simulink model "Observer_reconstruction"  (R2019b)
settings: Solver=ode1  StartTime=0.0  StopTime=5  FixedStep=0.002  RelTol=1e-3
values from neighbouring files (symbols this model uses):
  data = e_h.load_data    [potentiometer_recover.m]
undefined symbols (not defined in the file or in its folder): controller
settings Model: Creator=giacomo  LastModifiedBy=giacomo

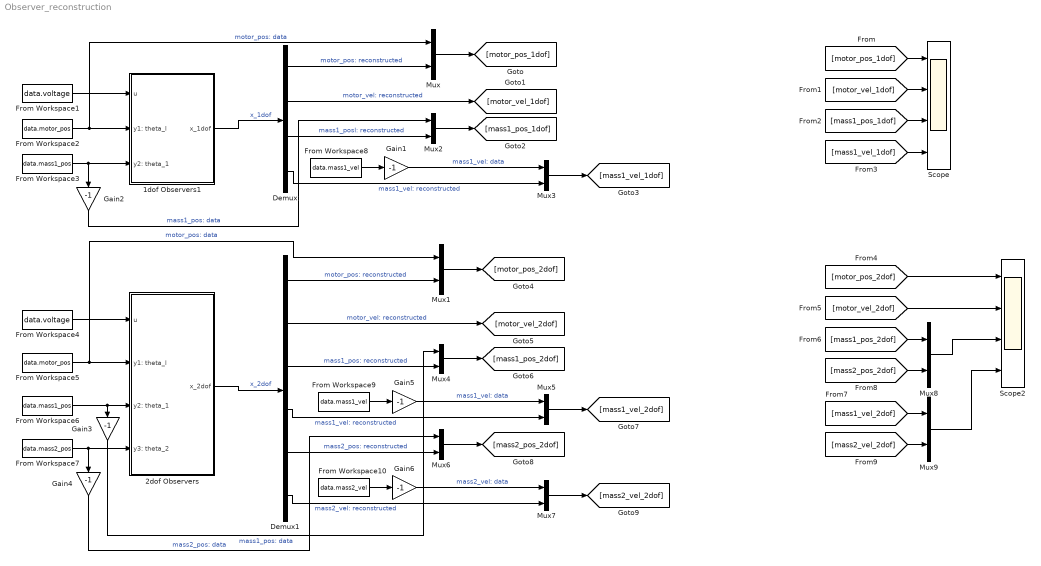
== system Observer_reconstruction ==
  1dof Observers1 : Subsystem
  2dof Observers : Subsystem
  Demux : Demux
  Demux1 : Demux  Outputs=6
  From Workspace1 : FromWorkspace  VariableName=data.voltage  SampleTime=0
  From Workspace10 : FromWorkspace  VariableName=data.mass2_vel  SampleTime=0
  From Workspace2 : FromWorkspace  VariableName=data.motor_pos  SampleTime=0
  From Workspace3 : FromWorkspace  VariableName=data.mass1_pos  SampleTime=0
  From Workspace4 : FromWorkspace  VariableName=data.voltage  SampleTime=0
  From Workspace5 : FromWorkspace  VariableName=data.motor_pos  SampleTime=0
  From Workspace6 : FromWorkspace  VariableName=data.mass1_pos  SampleTime=0
  From Workspace7 : FromWorkspace  VariableName=data.mass2_pos  SampleTime=0
  From Workspace8 : FromWorkspace  VariableName=data.mass1_vel  SampleTime=0
  From Workspace9 : FromWorkspace  VariableName=data.mass1_vel  SampleTime=0
  Gain{1..6} (6 alike) : Gain  Gain=-1
  Mux{,1..9} (10 alike) : Mux  Inputs=2
  Scope : Scope  NumInputPorts=4
  Scope2 : Scope  NumInputPorts=4
  wires:
  From Workspace2/1 -> Mux/1, 1dof Observers1/2(y1: theta_l)  "motor_pos: data"
  Demux/3 -> Mux2/2  "mass1_posl: reconstructed"
  1dof Observers1/1(x_1dof) -> Demux/1  "x_1dof"
  From Workspace1/1 -> 1dof Observers1/1(u)
  Demux/1 -> Mux/2  "motor_pos: reconstructed"
  Demux/4 -> Mux3/2  "mass1_vel: reconstructed"
  Mux/1 -> [motor_pos_1dof]
  Gain1/1 -> Mux3/1  "mass1_vel: data"
  From Workspace3/1 -> 1dof Observers1/3(y2: theta_1), Gain2/1
  Gain2/1 -> Mux2/1  "mass1_pos: data"
  [motor_pos_1dof] -> Scope/1
  Demux/2 -> [motor_vel_1dof]  "motor_vel: reconstructed"
  [motor_vel_1dof] -> Scope/2
  Mux2/1 -> [mass1_pos_1dof]
  Mux3/1 -> [mass1_vel_1dof]
  [mass1_pos_1dof] -> Scope/3
  [mass1_vel_1dof] -> Scope/4
  From Workspace8/1 -> Gain1/1
  From Workspace4/1 -> 2dof Observers/1("u ")
  From Workspace6/1 -> 2dof Observers/3(y2: theta_1), Gain3/1
  From Workspace7/1 -> 2dof Observers/4(y3: theta_2), Gain4/1
  Gain3/1 -> Mux4/1  "mass1_pos: data"
  2dof Observers/1(x_2dof) -> Demux1/1  "x_2dof"
  Mux5/1 -> [mass1_vel_2dof]
  Mux1/1 -> [motor_pos_2dof]
  From Workspace5/1 -> Mux1/1, 2dof Observers/2(y1: theta_l)  "motor_pos: data"
  Demux1/1 -> Mux1/2  "motor_pos: reconstructed"
  Demux1/3 -> Mux4/2  "mass1_pos: reconstructed"
  Demux1/4 -> Mux5/2  "mass1_vel: reconstructed"
  Mux4/1 -> [mass1_pos_2dof]
  Gain5/1 -> Mux5/1  "mass1_vel: data"
  Demux1/2 -> [motor_vel_2dof]  "motor_vel: reconstructed"
  From Workspace9/1 -> Gain5/1
  Mux7/1 -> [mass2_vel_2dof]
  Gain6/1 -> Mux7/1  "mass2_vel: data"
  From Workspace10/1 -> Gain6/1
  Demux1/5 -> Mux6/2  "mass2_pos: reconstructed"
  Demux1/6 -> Mux7/2  "mass2_vel: reconstructed"
  Mux6/1 -> [mass2_pos_2dof]
  Gain4/1 -> Mux6/1  "mass2_pos: data"
  [motor_pos_2dof] -> Scope2/1
  [motor_vel_2dof] -> Scope2/2
  [mass1_pos_2dof] -> Mux8/1
  [mass2_pos_2dof] -> Mux8/2
  Mux8/1 -> Scope2/3
  [mass2_vel_2dof] -> Mux9/2
  Mux9/1 -> Scope2/4
  [mass1_vel_2dof] -> Mux9/1

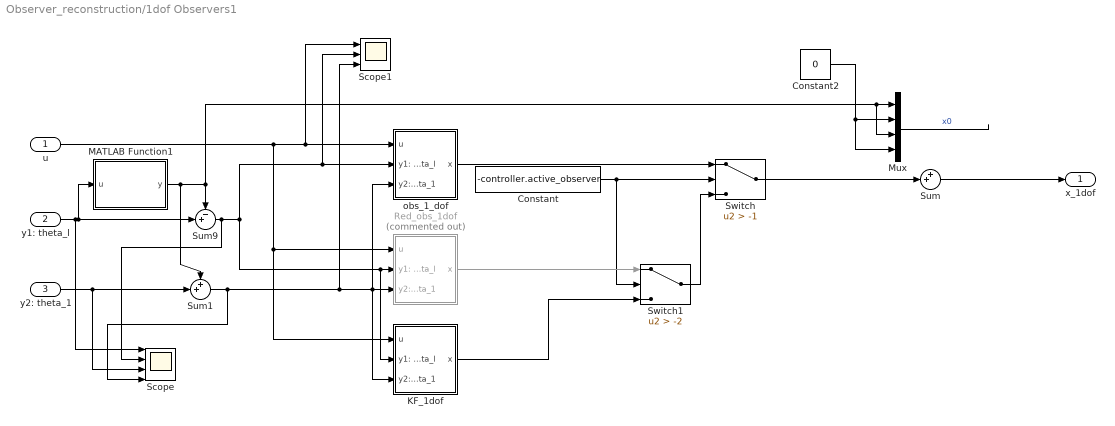
== system Observer_reconstruction/1dof Observers1 ==
  u : Inport
  y1: theta_l : Inport  Port=2
  y2: theta_1 : Inport  Port=3
  Constant : Constant  Value=-controller.active_observer
  Constant2 : Constant  Value=0
  KF_1dof : Subsystem
  MATLAB Function1 : MATLAB Function  TreatAsAtomicUnit=on  SystemSampleTime=0.002
  Mux : Mux
  Red_obs_1dof : Subsystem  Commented=on
  Scope : Scope  NumInputPorts=4
  Scope1 : Scope  NumInputPorts=3
  Sum : Sum  Inputs=++|
  Sum1 : Sum  Inputs=++|
  Sum9 : Sum  Inputs=-+|
  Switch : Switch  Criteria=u2 > Threshold  Threshold=-1
  Switch1 : Switch  Criteria=u2 > Threshold  Threshold=-2
  obs_1_dof : Subsystem
  x_1dof : Outport
  wires:
  Sum9/1 -> Scope/2, KF_1dof/2(y1: theta_l), Red_obs_1dof/2(y1: theta_l), Scope1/2, obs_1_dof/2(y1: theta_l)
  Sum1/1 -> Scope/4, Scope1/3, KF_1dof/3(y2: theta_1), obs_1_dof/3(y2: theta_1), Red_obs_1dof/3(y2: theta_1)
  Constant/1 -> Switch1/2, Switch/2
  u/1 -> Red_obs_1dof/1(u), KF_1dof/1(u), Scope1/1, obs_1_dof/1(u)
  Sum/1 -> x_1dof/1
  MATLAB Function1/1(y) -> Sum1/1, Sum9/1, Mux/3, Mux/1
  Mux/1 -> ?  "x0"
  Constant2/1 -> Mux/4, Mux/2
  Switch/1 -> Sum/2
  y1: theta_l/1 -> Scope/1, MATLAB Function1/1(u), Sum9/2
  obs_1_dof/1(x) -> Switch/1
  Red_obs_1dof/1(x) -> Switch1/1
  Switch1/1 -> Switch/3
  KF_1dof/1(x) -> Switch1/3
  y2: theta_1/1 -> Scope/3, Sum1/2

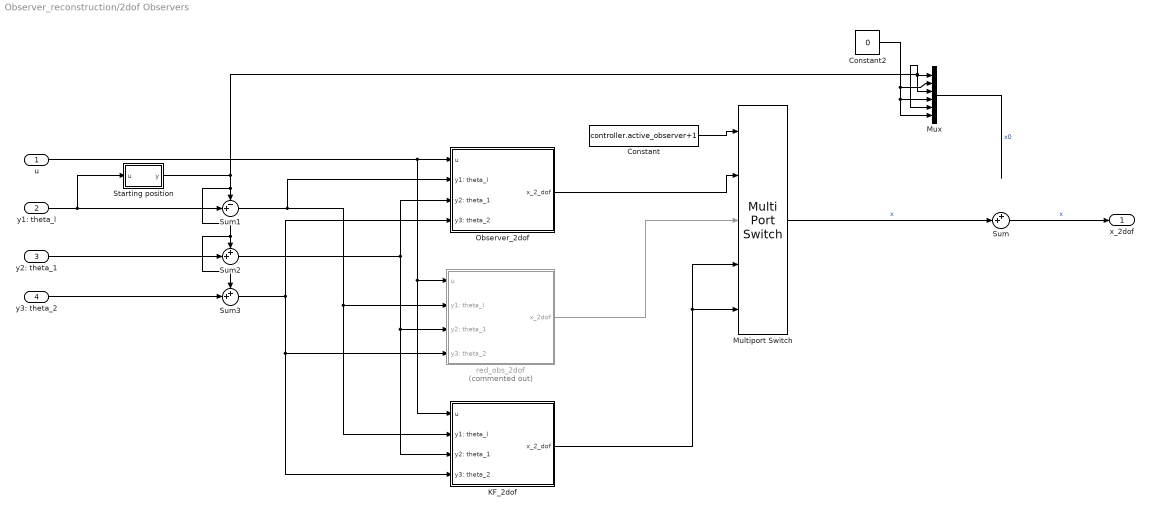
== system Observer_reconstruction/2dof Observers ==
  "u " : Inport
  y1: theta_l : Inport  Port=2
  y2: theta_1 : Inport  Port=3
  y3: theta_2 : Inport  Port=4
  Constant : Constant  Value=controller.active_observer+1
  Constant2 : Constant  Value=0
  KF_2dof : Subsystem
  Multiport Switch : MultiPortSwitch  Inputs=4
  Mux : Mux  Inputs=6
  Observer_2dof : Subsystem
  Starting position : MATLAB Function  TreatAsAtomicUnit=on  SystemSampleTime=0.002
  Sum : Sum  Inputs=++|
  Sum1 : Sum  Inputs=-+|
  Sum2 : Sum  Inputs=++|
  Sum3 : Sum  Inputs=++|
  red_obs_2dof : Subsystem  Commented=on
  x_2dof : Outport
  wires:
  Sum3/1 -> KF_2dof/4(y3: theta_2), red_obs_2dof/4(y3: theta_2), Observer_2dof/4(y3: theta_2)
  Sum2/1 -> KF_2dof/3(y2: theta_1), red_obs_2dof/3(y2: theta_1), Observer_2dof/3(y2: theta_1)
  "u "/1 -> KF_2dof/1(u), red_obs_2dof/1(u), Observer_2dof/1(u)
  Sum/1 -> x_2dof/1  "x"
  Starting position/1(y) -> Sum3/1, Sum2/1, Sum1/1, Mux/5, Mux/3, Mux/1
  Constant2/1 -> Mux/6, Mux/4, Mux/2
  Mux/1 -> ?  "x0"
  Sum1/1 -> KF_2dof/2(y1: theta_l), red_obs_2dof/2(y1: theta_l), Observer_2dof/2(y1: theta_l)
  y1: theta_l/1 -> Sum1/2, Starting position/1(u)
  Constant/1 -> Multiport Switch/1
  Observer_2dof/1(x_2_dof) -> Multiport Switch/2
  Multiport Switch/1 -> Sum/2  "x"
  y3: theta_2/1 -> Sum3/2
  y2: theta_1/1 -> Sum2/2
  red_obs_2dof/1(x_2dof) -> Multiport Switch/3
  KF_2dof/1(x_2_dof) -> Multiport Switch/5, Multiport Switch/4

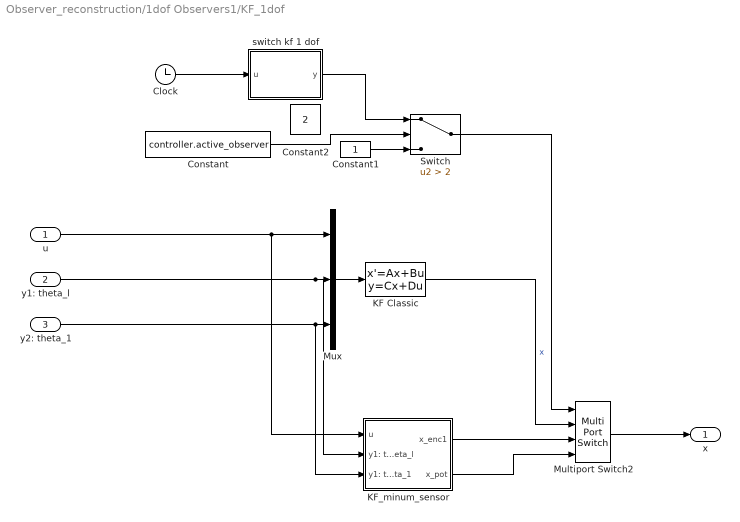
== system Observer_reconstruction/1dof Observers1/KF_1dof ==
  u : Inport
  y1: theta_l : Inport  Port=2
  y2: theta_1 : Inport  Port=3
  Clock : Clock
  Constant : Constant  Value=controller.active_observer
  Constant1 : Constant
  Constant2 : Constant  Value=2
  KF Classic : StateSpace  A=controller.KF_1dof.A  B=controller.KF_1dof.B  C=controller.KF_1dof.C  D=controller.KF_1dof.D  InitialCondition=[]
  KF_minum_sensor : Subsystem
  Multiport Switch2 : MultiPortSwitch
  Mux : Mux  Inputs=3
  Switch : Switch  Criteria=u2 > Threshold  Threshold=2
  switch kf 1 dof : MATLAB Function  TreatAsAtomicUnit=on
  x : Outport
  wires:
  Mux/1 -> KF Classic/1
  u/1 -> KF_minum_sensor/1(u), Mux/1
  y1: theta_l/1 -> KF_minum_sensor/2(y1: theta_l), Mux/2
  y2: theta_1/1 -> KF_minum_sensor/3(y1: theta_1), Mux/3
  KF Classic/1 -> Multiport Switch2/2  "x"
  Clock/1 -> switch kf 1 dof/1(u)
  Constant1/1 -> Switch/3
  switch kf 1 dof/1(y) -> Switch/1
  Constant/1 -> Switch/2
  Multiport Switch2/1 -> x/1
  KF_minum_sensor/1(x_enc1) -> Multiport Switch2/3
  KF_minum_sensor/2(x_pot) -> Multiport Switch2/4
  Switch/1 -> Multiport Switch2/1

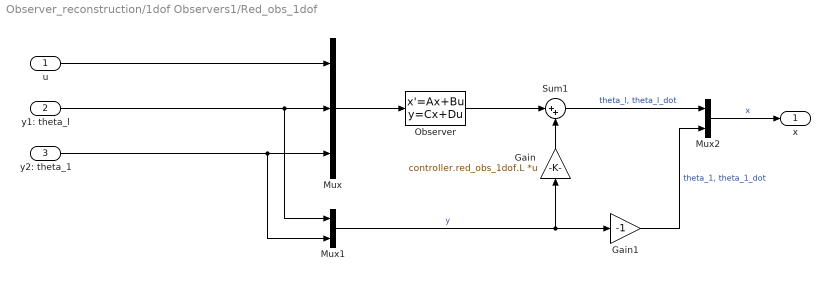
== system Observer_reconstruction/1dof Observers1/Red_obs_1dof ==
  u : Inport
  y1: theta_l : Inport  Port=2
  y2: theta_1 : Inport  Port=3
  Gain : Gain  Gain=controller.red_obs_1dof.L  Multiplication=Matrix(K*u)
  Gain1 : Gain  Gain=-1
  Mux : Mux  Inputs=3
  Mux1 : Mux  Inputs=2
  Mux2 : Mux  Inputs=2
  Observer : StateSpace  A=controller.red_obs_1dof.A  B=controller.red_obs_1dof.B  C=controller.red_obs_1dof.C  D=controller.red_obs_1dof.D  InitialCondition=[data.motor_pos_0;0]
  Sum1 : Sum  Inputs=|++
  x : Outport
  wires:
  Mux2/1 -> x/1  "x"
  u/1 -> Mux/1
  Gain1/1 -> Mux2/2  "theta_1, theta_1_dot"
  y2: theta_1/1 -> Mux/3, Mux1/2
  Gain/1 -> Sum1/2
  Mux1/1 -> Gain/1, Gain1/1  "y"
  y1: theta_l/1 -> Mux/2, Mux1/1
  Mux/1 -> Observer/1
  Sum1/1 -> Mux2/1  "theta_l, theta_l_dot"
  Observer/1 -> Sum1/1

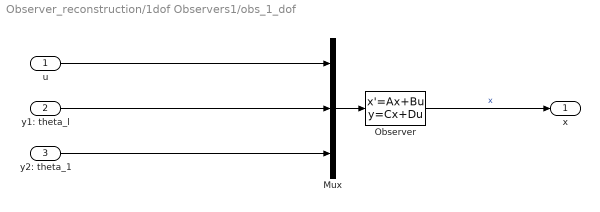
== system Observer_reconstruction/1dof Observers1/obs_1_dof ==
  u : Inport
  y1: theta_l : Inport  Port=2
  y2: theta_1 : Inport  Port=3
  Mux : Mux  Inputs=3
  Observer : StateSpace  A=controller.obs_1dof.A  B=controller.obs_1dof.B  C=controller.obs_1dof.C  D=controller.obs_1dof.D  InitialCondition=[]
  x : Outport
  wires:
  Mux/1 -> Observer/1
  u/1 -> Mux/1
  y1: theta_l/1 -> Mux/2
  y2: theta_1/1 -> Mux/3
  Observer/1 -> x/1  "x"

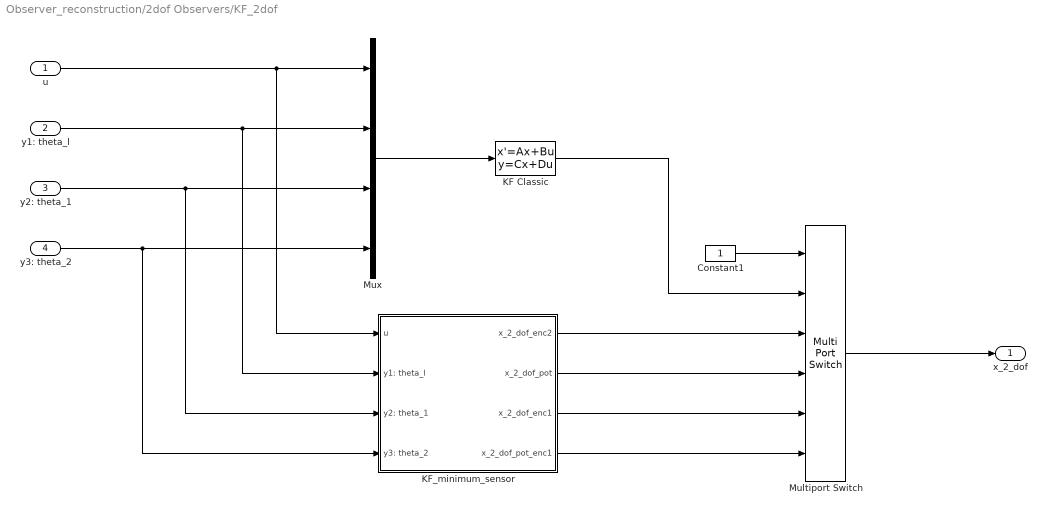
== system Observer_reconstruction/2dof Observers/KF_2dof ==
  u : Inport
  y1: theta_l : Inport  Port=2
  y2: theta_1 : Inport  Port=3
  y3: theta_2 : Inport  Port=4
  Constant1 : Constant
  KF Classic : StateSpace  A=controller.KF_2dof.A  B=controller.KF_2dof.B  C=controller.KF_2dof.C  D=controller.KF_2dof.D  InitialCondition=[]
  KF_minimum_sensor : Subsystem
  Multiport Switch : MultiPortSwitch  Inputs=5
  Mux : Mux
  x_2_dof : Outport
  wires:
  y1: theta_l/1 -> KF_minimum_sensor/2(y1: theta_l), Mux/2
  u/1 -> KF_minimum_sensor/1(u), Mux/1
  y3: theta_2/1 -> Mux/4, KF_minimum_sensor/4(y3: theta_2)
  Mux/1 -> KF Classic/1
  y2: theta_1/1 -> KF_minimum_sensor/3(y2: theta_1), Mux/3
  KF_minimum_sensor/1(x_2_dof_enc2) -> Multiport Switch/3
  KF_minimum_sensor/3(x_2_dof_enc1) -> Multiport Switch/5
  KF Classic/1 -> Multiport Switch/2
  KF_minimum_sensor/2(x_2_dof_pot) -> Multiport Switch/4
  Multiport Switch/1 -> x_2_dof/1
  KF_minimum_sensor/4(x_2_dof_pot_enc1) -> Multiport Switch/6
  Constant1/1 -> Multiport Switch/1

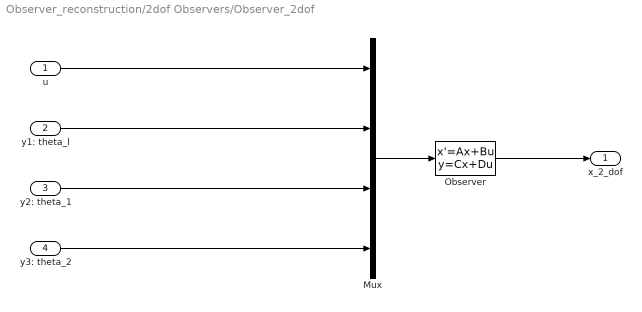
== system Observer_reconstruction/2dof Observers/Observer_2dof ==
  u : Inport
  y1: theta_l : Inport  Port=2
  y2: theta_1 : Inport  Port=3
  y3: theta_2 : Inport  Port=4
  Mux : Mux
  Observer : StateSpace  A=controller.obs_2dof.A  B=controller.obs_2dof.B  C=controller.obs_2dof.C  D=controller.obs_2dof.D  InitialCondition=[]
  x_2_dof : Outport
  wires:
  Observer/1 -> x_2_dof/1
  y1: theta_l/1 -> Mux/2
  u/1 -> Mux/1
  y3: theta_2/1 -> Mux/4
  Mux/1 -> Observer/1
  y2: theta_1/1 -> Mux/3

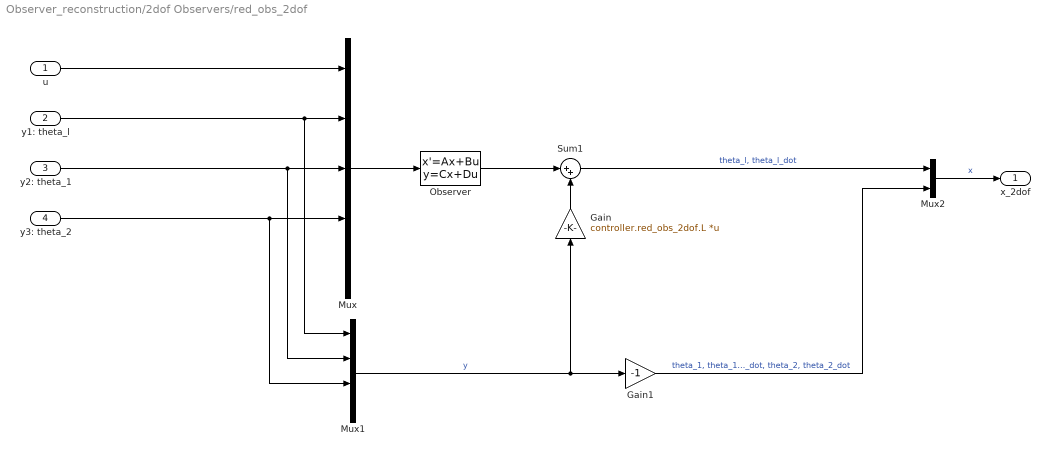
== system Observer_reconstruction/2dof Observers/red_obs_2dof ==
  u : Inport
  y1: theta_l : Inport  Port=2
  y2: theta_1 : Inport  Port=3
  y3: theta_2 : Inport  Port=4
  Gain : Gain  Gain=controller.red_obs_2dof.L  Multiplication=Matrix(K*u)
  Gain1 : Gain  Gain=-1
  Mux : Mux  Inputs=5
  Mux1 : Mux
  Mux2 : Mux  Inputs=2
  Observer : StateSpace  A=controller.red_obs_2dof.A  B=controller.red_obs_2dof.B  C=controller.red_obs_2dof.C  D=controller.red_obs_2dof.D  InitialCondition=[data.motor_pos_0;0]
  Sum1 : Sum  Inputs=|++
  x_2dof : Outport
  wires:
  Sum1/1 -> Mux2/1  "theta_l, theta_l_dot"
  y1: theta_l/1 -> Mux1/1, Mux/2
  Mux/1 -> Observer/1
  Observer/1 -> Sum1/1
  y2: theta_1/1 -> Mux1/2, Mux/3
  y3: theta_2/1 -> Mux1/3, Mux/4
  Mux1/1 -> Gain/1, Gain1/1  "y"
  u/1 -> Mux/1
  Gain/1 -> Sum1/2
  Gain1/1 -> Mux2/2  "theta_1, theta_1_dot, theta_2, theta_2_dot"
  Mux2/1 -> x_2dof/1  "x"

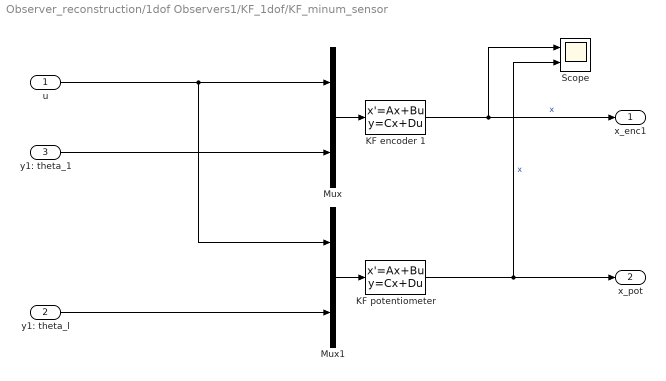
== system Observer_reconstruction/1dof Observers1/KF_1dof/KF_minum_sensor ==
  u : Inport
  y1: theta_l : Inport  Port=2
  y1: theta_1 : Inport  Port=3
  KF encoder 1 : StateSpace  A=controller.minKF_1dof_enc1.A  B=controller.minKF_1dof_enc1.B  C=controller.minKF_1dof_enc1.C  D=controller.minKF_1dof_enc1.D  InitialCondition=[]
  KF potentiometer : StateSpace  A=controller.minKF_1dof_pot.A  B=controller.minKF_1dof_pot.B  C=controller.minKF_1dof_pot.C  D=controller.minKF_1dof_pot.D  InitialCondition=[]
  Mux : Mux  Inputs=2
  Mux1 : Mux  Inputs=2
  Scope : Scope  NumInputPorts=2
  x_enc1 : Outport
  x_pot : Outport  Port=2
  wires:
  Mux/1 -> KF encoder 1/1
  y1: theta_1/1 -> Mux/2
  KF encoder 1/1 -> x_enc1/1, Scope/1  "x"
  u/1 -> Mux1/1, Mux/1
  y1: theta_l/1 -> Mux1/2
  Mux1/1 -> KF potentiometer/1
  KF potentiometer/1 -> x_pot/1, Scope/2  "x"

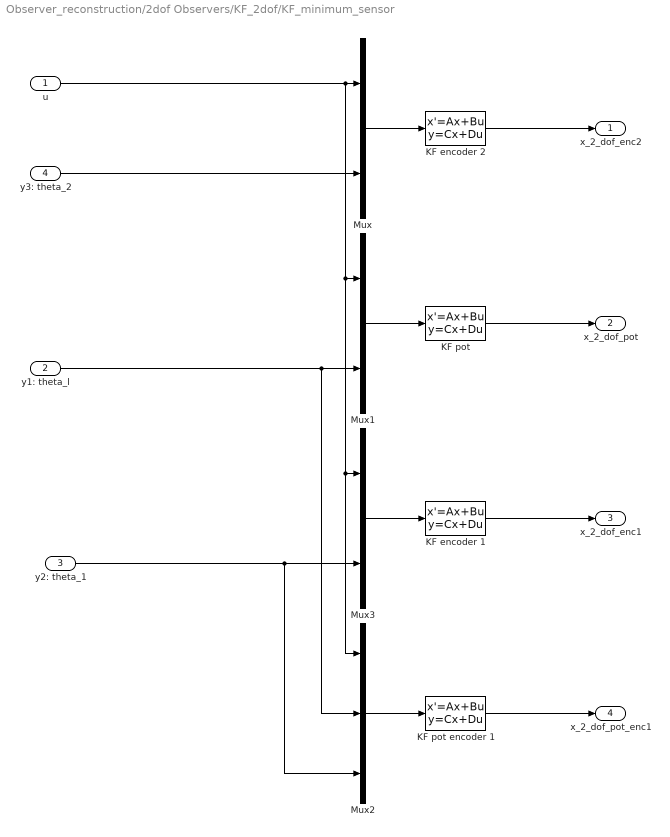
== system Observer_reconstruction/2dof Observers/KF_2dof/KF_minimum_sensor ==
  u : Inport
  y1: theta_l : Inport  Port=2
  y2: theta_1 : Inport  Port=3
  y3: theta_2 : Inport  Port=4
  KF encoder 1 : StateSpace  A=controller.minKF_2dof_enc1.A  B=controller.minKF_2dof_enc1.B  C=controller.minKF_2dof_enc1.C  D=controller.minKF_2dof_enc1.D  InitialCondition=[]
  KF encoder 2 : StateSpace  A=controller.minKF_2dof_enc2.A  B=controller.minKF_2dof_enc2.B  C=controller.minKF_2dof_enc2.C  D=controller.minKF_2dof_enc2.D  InitialCondition=[]
  KF pot : StateSpace  A=controller.minKF_2dof_pot.A  B=controller.minKF_2dof_pot.B  C=controller.minKF_2dof_pot.C  D=controller.minKF_2dof_pot.D  InitialCondition=[]
  KF pot encoder 1 : StateSpace  A=controller.minKF_2dof_potenc1.A  B=controller.minKF_2dof_potenc1.B  C=controller.minKF_2dof_potenc1.C  D=controller.minKF_2dof_potenc1.D  InitialCondition=[]
  Mux : Mux  Inputs=2
  Mux1 : Mux  Inputs=2
  Mux2 : Mux  Inputs=3
  Mux3 : Mux  Inputs=2
  x_2_dof_enc2 : Outport
  x_2_dof_pot : Outport  Port=2
  x_2_dof_enc1 : Outport  Port=3
  x_2_dof_pot_enc1 : Outport  Port=4
  wires:
  y3: theta_2/1 -> Mux/2
  u/1 -> Mux2/1, Mux3/1, Mux1/1, Mux/1
  Mux/1 -> KF encoder 2/1
  Mux2/1 -> KF pot encoder 1/1
  Mux3/1 -> KF encoder 1/1
  Mux1/1 -> KF pot/1
  y1: theta_l/1 -> Mux1/2, Mux2/2
  y2: theta_1/1 -> Mux3/2, Mux2/3
  KF encoder 2/1 -> x_2_dof_enc2/1
  KF encoder 1/1 -> x_2_dof_enc1/1
  KF pot/1 -> x_2_dof_pot/1
  KF pot encoder 1/1 -> x_2_dof_pot_enc1/1

== matlab function Observer_reconstruction/1dof Observers1/KF_1dof/switch kf 1 dof ==
  data: u input; y output
function y = fcn(u)
if u < 15
    % kf classic
    y = 1;
elseif u <30 
    % kf enc 1
    y = 2;
elseif u < 45
    %kf pot
    y = 3;
else
    y = 1;
end

== matlab function Observer_reconstruction/1dof Observers1/MATLAB Function1 ==
  data: u input; y output
function y = fcn(u)
persistent oldu
if isempty(oldu) 
    oldu = u;
end
y = oldu;

== matlab function Observer_reconstruction/2dof Observers/Starting position ==
  data: u input; y output
function y = fcn(u)
persistent oldu
if isempty(oldu) 
    oldu = u;
end
y = oldu;
